simulink model "Exercise_1"  (R2020b)
settings: Solver=VariableStepAuto  StartTime=0.0  StopTime=10.0  RelTol=1e-3
libraries: fl_lib x13, nesl_utility x3
settings Model: Creator=zaliyazici  LastModifiedBy=zaliyazici

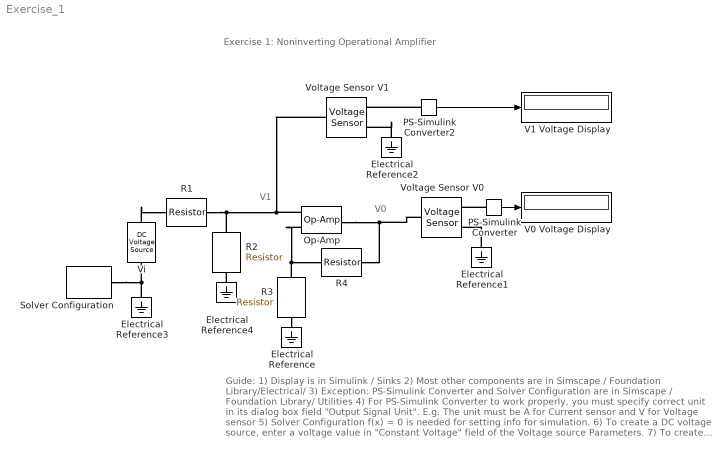
== system Exercise_1 ==
  note: V0
  note: Guide:
      | 1) Display is in Simulink / Sinks
      | 2) Most other components are in Simscape / Foundation Library/Electrical/
      | 3) Exception: PS-Simulink Converter and Solver Configuration are in Simscape / Foundation Library/ Utilities
      | 4) For PS-Simulink Converter to work properly, you must specify correct unit in its dialog box field "Output Signal Unit".
      | E.g. The unit must be A for Current sensor and V for Voltage sensor
      | 5) Solver Configuration f(x) = 0 is needed for setting info for simulation.
      | 6) To create a DC voltage source, enter a voltage value in "Constant Voltage" field of the Voltage source Parameters.
      | 7) To create "Annotation", double-click a location on project page and select "Create annotation" from the prompt. Then, type any text you want to clarify your circuit. E.g. "Display for Current".
      | 8) To understand how to use a component, right-click on the component and select "Help".
      | Measurement: Node voltages V1 and V0
  note: Exercise 1: Noninverting Operational Amplifier
  note: V1
  Electrical Reference{,1..4} (5 alike) : fl_lib/Electrical/Electrical Elements/Electrical Reference
  Op-Amp : fl_lib/Electrical/Electrical Elements/Op-Amp  outI_specify=off  outI_priority=None  outI=0 A  outI_nominal_specify=off  outI_nominal_unit=A  outI_nominal_value=1
  PS-Simulink Converter : nesl_utility/PS-Simulink Converter  PhysicalDomain=network_engine_domain  SubClassName=ps_output  LeftPortType=input  RightPortType=output  PseudoPeriodic=off  Frequencies=[]  Unit=V  AffineConversion=off
  PS-Simulink Converter2 : nesl_utility/PS-Simulink Converter  PhysicalDomain=network_engine_domain  SubClassName=ps_output  LeftPortType=input  RightPortType=output  PseudoPeriodic=off  Frequencies=[]  Unit=V  AffineConversion=off
  R1 : fl_lib/Electrical/Electrical Elements/Resistor  R=1 kOhm  i_specify=off  i_priority=None  i=0 A  i_nominal_specify=off  i_nominal_unit=A  i_nominal_value=1  v_specify=off  v_priority=None  v=0 V  v_nominal_specify=off  v_nominal_unit=V  v_nominal_value=1
      settings: AttributesFormatString=%<R> %<R_unit>  LogSimulationData=on
  R2 : fl_lib/Electrical/Electrical Elements/Resistor  R=4 kOhm  i_specify=off  i_priority=None  i=0 A  i_nominal_specify=off  i_nominal_unit=A  i_nominal_value=1  v_specify=off  v_priority=None  v=0 V  v_nominal_specify=off  v_nominal_unit=V  v_nominal_value=1
      settings: AttributesFormatString=%<R> %<R_unit>  LogSimulationData=on
  R3 : fl_lib/Electrical/Electrical Elements/Resistor  R=4 kOhm  i_specify=off  i_priority=None  i=0 A  i_nominal_specify=off  i_nominal_unit=A  i_nominal_value=1  v_specify=off  v_priority=None  v=0 V  v_nominal_specify=off  v_nominal_unit=V  v_nominal_value=1
      settings: AttributesFormatString=%<R> %<R_unit>  LogSimulationData=on
  R4 : fl_lib/Electrical/Electrical Elements/Resistor  R=5 kOhm  i_specify=off  i_priority=None  i=0 A  i_nominal_specify=off  i_nominal_unit=A  i_nominal_value=1  v_specify=off  v_priority=None  v=0 V  v_nominal_specify=off  v_nominal_unit=V  v_nominal_value=1
      settings: AttributesFormatString=%<R> %<R_unit>  LogSimulationData=on
  Solver Configuration : nesl_utility/Solver Configuration  PhysicalDomain=network_engine_domain  SubClassName=solver  LeftPortType=input  RightPortType=generic  Tones=[]  Harmonics=[]  SimulateNoise=off  Profile=off  UseLocalSampling=off  EnableSwitchedLinearOptims=on  FrequencyDomain=off  UseCCode=off  RelTol=0.001  AbsTol=1e-06  MinStep=1e-09  ToWorkspace=off  RevertToSquareIcSolve=off  NumHomotopyIterations=100  PhasorMode=off  PhasorModeNumHarmonics=1  DoDC=off  ResidualTolerance=1e-09  UseLocalSolver=off  LocalSolverChoice=NE_BACKWARD_EULER_ADVANCER  LocalSolverSampleTime=0.001  DoFixedCost=off  MaxNonlinIter=3  MaxModeIter=2  ComputeImpulses=off  ImpulseIterations=2  LinearAlgebra=auto  EquationFormulation=NE_TIME_EF  DelaysMemoryBudget=1024  AutomaticFiltering=on  FilteringTimeConstant=0.001  PartitionStorageMethod=AS_NEEDED  PartitionMemoryBudget=1024  PartitionMethod=ROBUST
  V0 Voltage Display : Display
  V1 Voltage Display : Display
  Vi : fl_lib/Electrical/Electrical Sources/DC Voltage Source  v0=2 V
      settings: AttributesFormatString=%<v0> %<v0_unit>
  Voltage Sensor V0 : fl_lib/Electrical/Electrical Sensors/Voltage Sensor
  Voltage Sensor V1 : fl_lib/Electrical/Electrical Sensors/Voltage Sensor
  wires:
  PS-Simulink Converter/1 -> V0 Voltage Display/1
  PS-Simulink Converter2/1 -> V1 Voltage Display/1
  connections:
  Vi/LConn1 -- R1/LConn1
  R3/RConn1 -- Electrical Reference/LConn1
  Electrical Reference1/LConn1 -- Voltage Sensor V0/RConn2
  PS-Simulink Converter/LConn1 -- Voltage Sensor V0/RConn1
  PS-Simulink Converter2/LConn1 -- Voltage Sensor V1/RConn1
  R1/RConn1 -- Voltage Sensor V1/LConn1 -- Op-Amp/LConn2 -- R2/LConn1
  Op-Amp/RConn1 -- R4/LConn1 -- Voltage Sensor V0/LConn1
  Electrical Reference2/LConn1 -- Voltage Sensor V1/RConn2
  Op-Amp/LConn1 -- R4/RConn1 -- R3/LConn1
  Solver Configuration/RConn1 -- Electrical Reference3/LConn1 -- Vi/RConn1
  Electrical Reference4/LConn1 -- R2/RConn1
